simulink model "Nelinearni_system_s_regulatorem"  (R2020a)
settings: Solver=VariableStepAuto  StartTime=0.0  StopTime=50  RelTol=1e-3
values from neighbouring files (symbols this model uses):
  dphi = 0    [Model_kyvadla_na_voziku_m.m]
  dx = 0    [Model_kyvadla_na_voziku_m.m]
  f = 0    [Model_kyvadla_na_voziku_m.m]
  g = 9.81    [Model_kyvadla_na_voziku_m.m]
  K = acker(sys.A, sys.B, [p1, p2, p3, p4])    [Model_kyvadla_na_voziku_m.m]
  l = 1    [Model_kyvadla_na_voziku_m.m]
  m = 5    [Model_kyvadla_na_voziku_m.m]
  M = 15    [Model_kyvadla_na_voziku_m.m]
  phi = deg2rad(5)    [Model_kyvadla_na_voziku_m.m]
  x = 0    [Model_kyvadla_na_voziku_m.m]
settings Model: Creator=Jiří  LastModifiedBy=Jiří

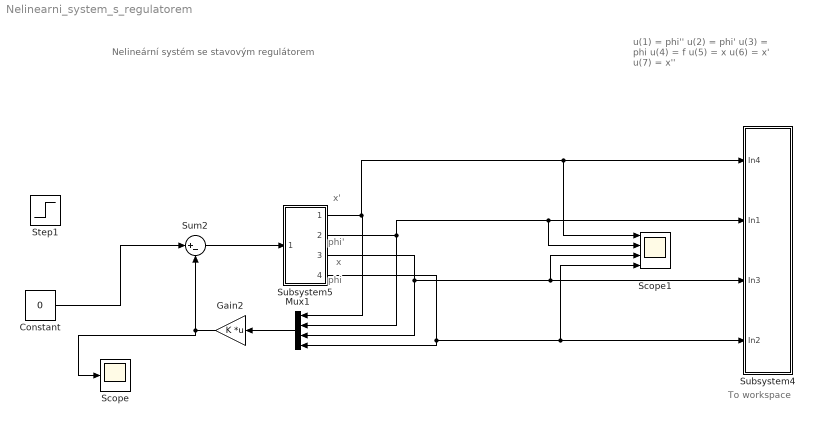
== system Nelinearni_system_s_regulatorem ==
  note: x
  note: x'
  note: phi'
  note: u(1) = phi''
      | u(2) = phi'
      | u(3) = phi
      | u(4) = f
      | u(5) = x
      | u(6) = x'
      | u(7) = x''
  note: Nelineární systém se stavovým regulátorem
  note: To workspace
  note: phi
  Constant : Constant  Value=0
  Gain2 : Gain  Gain=K  Multiplication=Matrix(K*u)
  Mux1 : Mux
  Scope : Scope
  Scope1 : Scope  NumInputPorts=4
  Step1 : Step  Time=10  After=f  SampleTime=1
  Subsystem4 : Subsystem
  Subsystem5 : Subsystem
  Sum2 : Sum  Inputs=|+-
  wires:
  Sum2/1 -> Subsystem5/1(In1)
  Subsystem5/1(Out4) -> Scope1/1, Subsystem4/1(In4), Mux1/1
  Gain2/1 -> Scope/1, Sum2/2
  Subsystem5/4(Out2) -> Mux1/4, Scope1/4, Subsystem4/4(In2)
  Mux1/1 -> Gain2/1
  Subsystem5/2(Out1) -> Mux1/2, Scope1/2, Subsystem4/2(In1)
  Subsystem5/3(Out3) -> Mux1/3, Scope1/3, Subsystem4/3(In3)
  Constant/1 -> Sum2/1

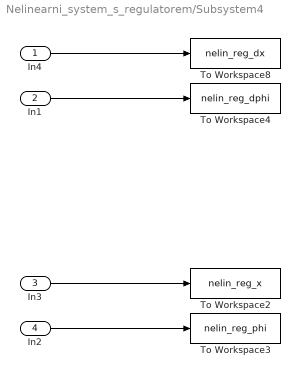
== system Nelinearni_system_s_regulatorem/Subsystem4 ==
  In4 : Inport
  In1 : Inport  Port=2
  In3 : Inport  Port=3
  In2 : Inport  Port=4
  To Workspace2 : ToWorkspace  VariableName=nelin_reg_x  SaveFormat=Timeseries  SampleTime=-1
  To Workspace3 : ToWorkspace  VariableName=nelin_reg_phi  SaveFormat=Timeseries  SampleTime=-1
  To Workspace4 : ToWorkspace  VariableName=nelin_reg_dphi  SaveFormat=Timeseries  SampleTime=-1
  To Workspace8 : ToWorkspace  VariableName=nelin_reg_dx  SaveFormat=Timeseries  SampleTime=-1
  wires:
  In1/1 -> To Workspace4/1
  In2/1 -> To Workspace3/1
  In3/1 -> To Workspace2/1
  In4/1 -> To Workspace8/1

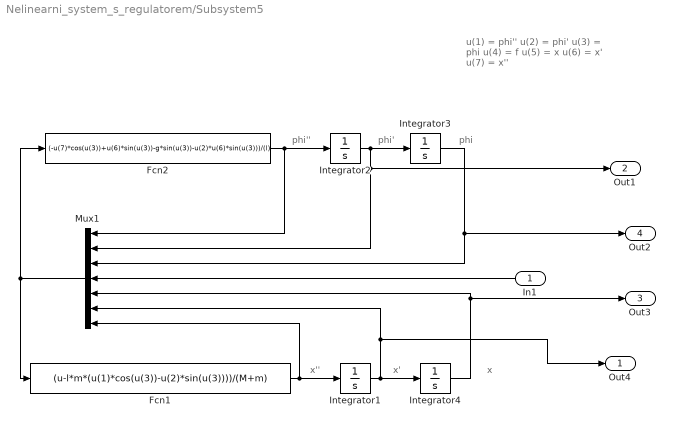
== system Nelinearni_system_s_regulatorem/Subsystem5 ==
  note: x''
  note: x'
  note: x
  note: phi''
  note: phi'
  note: phi
  note: u(1) = phi''
      | u(2) = phi'
      | u(3) = phi
      | u(4) = f
      | u(5) = x
      | u(6) = x'
      | u(7) = x''
  In1 : Inport
  Fcn1 : Fcn  Expr=(u-l*m*(u(1)*cos(u(3))-u(2)*sin(u(3))))/(M+m)
  Fcn2 : Fcn  Expr=(-u(7)*cos(u(3))+u(6)*sin(u(3))-g*sin(u(3))-u(2)*u(6)*sin(u(3)))/(l)
  Integrator1 : Integrator  InitialCondition=dx
  Integrator2 : Integrator  InitialCondition=dphi
  Integrator3 : Integrator  InitialCondition=phi
  Integrator4 : Integrator  InitialCondition=x
  Mux1 : Mux  Inputs=7
  Out4 : Outport
  Out1 : Outport  Port=2
  Out3 : Outport  Port=3
  Out2 : Outport  Port=4
  wires:
  Integrator1/1 -> Out4/1, Mux1/6, Integrator4/1
  Fcn2/1 -> Integrator2/1, Mux1/1
  Fcn1/1 -> Integrator1/1, Mux1/7
  Integrator3/1 -> Out2/1, Mux1/3
  Integrator4/1 -> Out3/1, Mux1/5
  Mux1/1 -> Fcn1/1, Fcn2/1
  Integrator2/1 -> Out1/1, Mux1/2, Integrator3/1
  In1/1 -> Mux1/4
